simulink model "AMCLIB_FW_BAM_F16"  (Simulink 8.3)
settings: Solver=ode45  StartTime=0.0  StopTime=10.0  RelTol=1e-3
undefined symbols (not defined in the file): f16IntegGainFW, f16PropGainFW, s16IntegGainShiftFW, s16PropGainShiftFW, u16NSamplesFW
settings Model: Creator=B37097  LastModifiedBy=B37097
settings DataIOCC: SignalLoggingSaveFormat=Dataset
settings DebuggingCC: UnderspecifiedInitializationDetection=Simplified  StateNameClashWarn=none
settings GRTTargetCC: CombineOutputUpdateFcns=on  GRTInterface=off

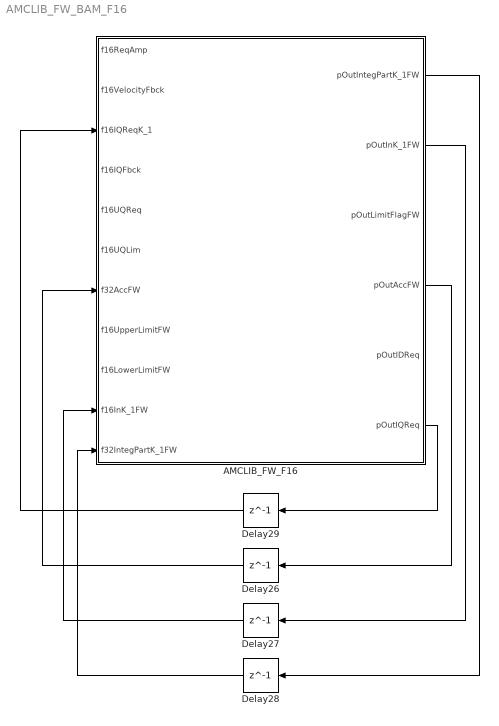
== system AMCLIB_FW_BAM_F16 ==
  AMCLIB_FW_F16 : Subsystem  mask(AMCLIB_FW_F16){u16NSamplesFW=u16NSamplesFW, f16PropGainFW=f16PropGainFW, s16PropGainShiftFW=s16PropGainShiftFW, f16IntegGainFW=f16IntegGainFW, s16IntegGainShiftFW=s16IntegGainShiftFW}
      mask help: Bit accurate model of the speed loop algorithm with field weakening capability in 16-bit fixed-point implementation.
      mask init:
      | pos = get_param(gcb, 'Position');width = pos(3) - pos(1); height = pos(4) - pos(2);tX=width/2;tY=height*0.9;
      mask Display: color('black');port_label('input',1,'f16ReqAmp');port_label('input',2,'f16VelocityFbck');port_label('input',3,'f16IQReqK_1');port_label('input',4,'f16IQFbck');port_label('input',5,'f16UQReq');port_label('input',6,'f16UQLim');port_label('input',7,'f32AccFW');port_label('input',8,'f16UpperLimitFW');port_label('input',9,'f16LowerLimitFW');port_label('input',10,'f16InK_1FW');port_label('input',11,'f32IntegPartK_1FW');port_label('output',1,'pOutIntegPartK_1FW');port_label('output',2,'pOutInK_1FW');port_label('output',3,'pOutLimitFlagFW');port_label('output',4,'pOutAccFW');port_label('output',5,'pOutIDReq');port_label('output',6,'pOutIQReq');color('black');disp('AMCLIB_FW_F16');color('blue');text(tX,tY, 'BAM', 'horizontalAlignment', 'center');
  Delay{26..29} (4 alike) : Delay  DelayLength=1  InitialCondition=0
  wires:
  AMCLIB_FW_F16/6(pOutIQReq) -> Delay29/1
  Delay29/1 -> AMCLIB_FW_F16/3(f16IQReqK_1)
  AMCLIB_FW_F16/4(pOutAccFW) -> Delay26/1
  AMCLIB_FW_F16/2(pOutInK_1FW) -> Delay27/1
  AMCLIB_FW_F16/1(pOutIntegPartK_1FW) -> Delay28/1
  Delay28/1 -> AMCLIB_FW_F16/11(f32IntegPartK_1FW)
  Delay27/1 -> AMCLIB_FW_F16/10(f16InK_1FW)
  Delay26/1 -> AMCLIB_FW_F16/7(f32AccFW)

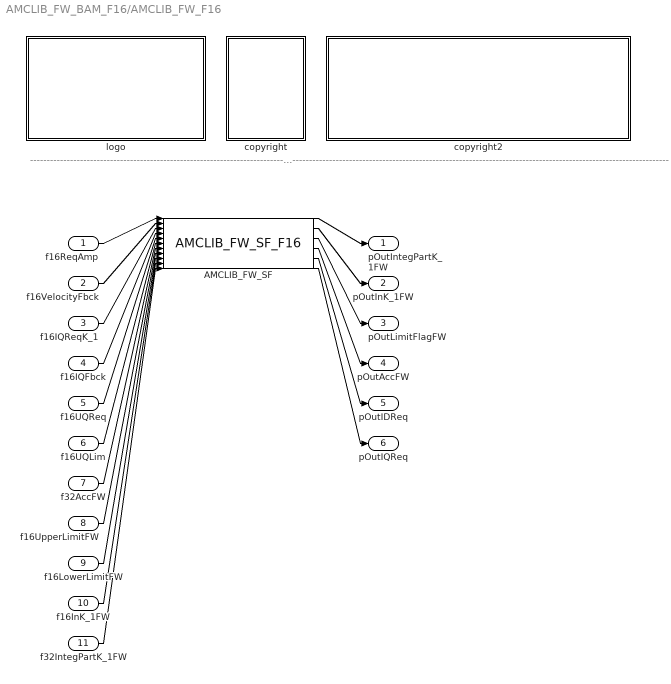
== system AMCLIB_FW_BAM_F16/AMCLIB_FW_F16 ==
  note: ---------------------------------------------------------------------------------------------------------------------------------------------------------------------------------------------------
  f16ReqAmp : Inport
  f16VelocityFbck : Inport  Port=2
  f16IQReqK_1 : Inport  Port=3
  f16IQFbck : Inport  Port=4
  f16UQReq : Inport  Port=5
  f16UQLim : Inport  Port=6
  f32AccFW : Inport  Port=7
  f16UpperLimitFW : Inport  Port=8
  f16LowerLimitFW : Inport  Port=9
  f16InK_1FW : Inport  Port=10
  f32IntegPartK_1FW : Inport  Port=11
  AMCLIB_FW_SF : S-Function  FunctionName=AMCLIB_FW_SF_F16  Parameters=u16NSamplesFW,f16PropGainFW,s16PropGainShiftFW,f16IntegGainFW,s16IntegGainShiftFW  EnableBusSupport=off
  copyright : Subsystem
      mask Display: text(10,90,'FILE:');text(10,75,'DESRIPTION:');text(10,60,'COPYRIGHT:');text(10,45,'VERSION:');text(10,30,'DATE:')
  copyright2 : Subsystem
      mask Display: text(10,90,'AMCLIB_FW_BAM_F16.mdl');text(10,75,'Speed Loop with Field Weakening.');text(10,60,'NXP');text(10,45,'1.0');text(10,30,'28-Aug-2017');
  logo : Subsystem
      mask Display: image(imread('logo.jpg'))
  pOutIntegPartK_1FW : Outport
  pOutInK_1FW : Outport  Port=2
  pOutLimitFlagFW : Outport  Port=3
  pOutAccFW : Outport  Port=4
  pOutIDReq : Outport  Port=5
  pOutIQReq : Outport  Port=6
  wires:
  f16ReqAmp/1 -> AMCLIB_FW_SF/1
  f16VelocityFbck/1 -> AMCLIB_FW_SF/2
  f16IQReqK_1/1 -> AMCLIB_FW_SF/3
  f16IQFbck/1 -> AMCLIB_FW_SF/4
  f16UQReq/1 -> AMCLIB_FW_SF/5
  f16UQLim/1 -> AMCLIB_FW_SF/6
  f32AccFW/1 -> AMCLIB_FW_SF/7
  f16UpperLimitFW/1 -> AMCLIB_FW_SF/8
  f16LowerLimitFW/1 -> AMCLIB_FW_SF/9
  f16InK_1FW/1 -> AMCLIB_FW_SF/10
  f32IntegPartK_1FW/1 -> AMCLIB_FW_SF/11
  AMCLIB_FW_SF/1 -> pOutIntegPartK_1FW/1
  AMCLIB_FW_SF/2 -> pOutInK_1FW/1
  AMCLIB_FW_SF/3 -> pOutLimitFlagFW/1
  AMCLIB_FW_SF/4 -> pOutAccFW/1
  AMCLIB_FW_SF/5 -> pOutIDReq/1
  AMCLIB_FW_SF/6 -> pOutIQReq/1

== system AMCLIB_FW_BAM_F16/AMCLIB_FW_F16/copyright ==

== system AMCLIB_FW_BAM_F16/AMCLIB_FW_F16/copyright2 ==

== system AMCLIB_FW_BAM_F16/AMCLIB_FW_F16/logo ==
